simulink model "W1"  (R2017b)
settings: Solver=FixedStepDiscrete  StartTime=0.0  StopTime=10.0  FixedStep=0.200000  RelTol=1e-3
libraries: sldvlib x2
settings Model: Creator=hbourbou  LastModifiedBy=hbourbou
settings OptimizationCC: LifeSpan=inf
settings DebuggingCC: SFExecutionAtInitializationDiag=none
settings HardwareCC: ProdBitPerSizeT=32  ProdBitPerPtrDiffT=32  ProdWordSize=32  ProdHWDeviceType=Specified
settings CodeAppCC: StateflowObjectComments=on

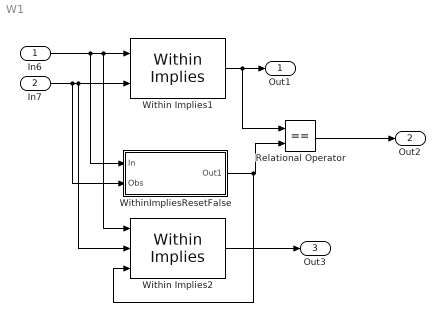
== system W1 ==
  In6 : Inport  OutDataTypeStr=boolean
  In7 : Inport  Port=2  OutDataTypeStr=boolean
  Relational Operator : RelationalOperator  Operator===  OutDataTypeStr=boolean  RndMeth=Nearest
  Within Implies1 : sldvlib/Temporal Operators/Within Implies  reset=off
      settings: SourceProductName=Simulink Design Verifier  SourceProductBaseCode=DV
  Within Implies2 : sldvlib/Temporal Operators/Within Implies  reset=on
      settings: SourceProductName=Simulink Design Verifier  SourceProductBaseCode=DV
  WithinImpliesResetFalse : Subsystem  mask(Within Implies){reset=off}
      mask prompts: reset "External reset"
      mask Display:
      | color('gray');
      |  plot([0.19 0.23 0.23 4.000000e-01 4.000000e-01 5.000000e-01 5.000000e-01 6.000000e-01 6.000000e-01 0.75],[ 7.000000e-01 7.000000e-01 8.500000e-01 8.500000e-01 7.000000e-01 7.000000e-01 8.500000e-01 8.500000e-01 7.000000e-01 7.000000e-01]);
      |  color('gray');
      |  plot([0.19 0.3 0.3 0.35 0.35 0.75],[ 5.600000e-01 5.600000e-01 7.100000e-01 7.100000e-01 5.600000e-01 5.600000e-01]);
      |  color('black');
      |  plot([0.19 6.000000e-01 6.000000e-01 6.200000e-01 6.200000e-01 0.75], [3.700000e-01, 3.700000e-01 2.200000e-01 2.200000e-01 3.700000e-01 3.700000e-01]);
  Out1 : Outport
  Out2 : Outport  Port=2
  Out3 : Outport  Port=3
  wires:
  In6/1 -> WithinImpliesResetFalse/1(In), Within Implies2/1, Within Implies1/1
  In7/1 -> WithinImpliesResetFalse/2(Obs), Within Implies2/2, Within Implies1/2
  Within Implies1/1 -> Relational Operator/1, Out1/1
  WithinImpliesResetFalse/1(Out1) -> Within Implies2/3, Relational Operator/2
  Relational Operator/1 -> Out2/1
  Within Implies2/1 -> Out3/1

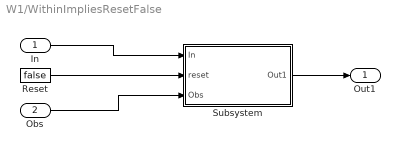
== system W1/WithinImpliesResetFalse ==
  In : Inport  OutDataTypeStr=boolean
  Obs : Inport  Port=2  OutDataTypeStr=boolean
  Reset : Constant  Value=false
  Subsystem : Subsystem
  Out1 : Outport
  wires:
  In/1 -> Subsystem/1(In)
  Reset/1 -> Subsystem/2(reset)
  Obs/1 -> Subsystem/3(Obs)
  Subsystem/1(Out1) -> Out1/1

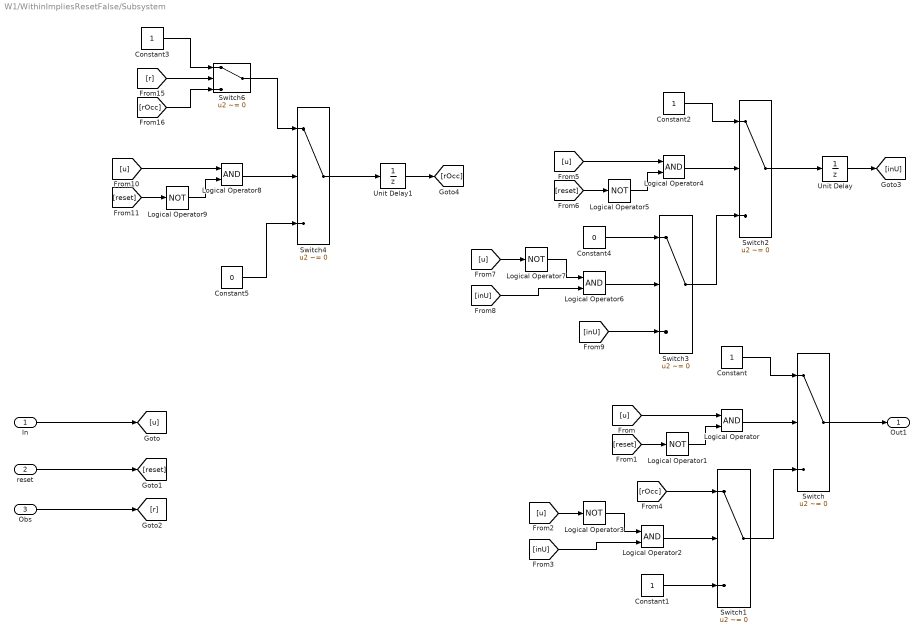
== system W1/WithinImpliesResetFalse/Subsystem ==
  In : Inport  OutDataTypeStr=boolean
  reset : Inport  Port=2
  Obs : Inport  Port=3  OutDataTypeStr=boolean
  Constant{,1..3} (4 alike) : Constant  OutDataTypeStr=boolean
  Constant4 : Constant  Value=0  OutDataTypeStr=boolean
  Constant5 : Constant  Value=0  OutDataTypeStr=boolean
  Logical Operator{,2,4,6,8} (5 alike) : Logic  AllPortsSameDT=off  OutDataTypeStr=boolean
  Logical Operator{1,3,5,7,9} (5 alike) : Logic  Operator=NOT  AllPortsSameDT=off  OutDataTypeStr=boolean
  Switch{,1..4,6} (6 alike) : Switch  Criteria=u2 ~= 0
  Unit Delay : UnitDelay  SampleTime=-1
  Unit Delay1 : UnitDelay  SampleTime=-1
  Out1 : Outport
  wires:
  reset/1 -> [reset]
  In/1 -> [u]
  Obs/1 -> [r]
  Unit Delay/1 -> [inU]
  Unit Delay1/1 -> [rOcc]
  Switch/1 -> Out1/1
  Logical Operator/1 -> Switch/2
  [u] -> Logical Operator/1
  Logical Operator1/1 -> Logical Operator/2
  [reset] -> Logical Operator1/1
  Constant/1 -> Switch/1
  Switch1/1 -> Switch/3
  Logical Operator2/1 -> Switch1/2
  Logical Operator3/1 -> Logical Operator2/1
  [u] -> Logical Operator3/1
  [inU] -> Logical Operator2/2
  [rOcc] -> Switch1/1
  Constant1/1 -> Switch1/3
  [reset] -> Logical Operator5/1
  [u] -> Logical Operator7/1
  Logical Operator5/1 -> Logical Operator4/2
  Constant2/1 -> Switch2/1
  Logical Operator4/1 -> Switch2/2
  [inU] -> Switch3/3
  Logical Operator6/1 -> Switch3/2
  [u] -> Logical Operator4/1
  Constant4/1 -> Switch3/1
  Switch3/1 -> Switch2/3
  Logical Operator7/1 -> Logical Operator6/1
  [inU] -> Logical Operator6/2
  Switch2/1 -> Unit Delay/1
  [u] -> Logical Operator8/1
  [reset] -> Logical Operator9/1
  Constant5/1 -> Switch4/3
  Logical Operator8/1 -> Switch4/2
  Logical Operator9/1 -> Logical Operator8/2
  Switch4/1 -> Unit Delay1/1
  Switch6/1 -> Switch4/1
  [r] -> Switch6/2
  Constant3/1 -> Switch6/1
  [rOcc] -> Switch6/3
